simulink model "Test_N3"  (R2022a)
settings: Solver=ode3  StartTime=0.0  StopTime=inf  FixedStep=0.05  RelTol=1e-3
libraries: EcBlockToolbox x1

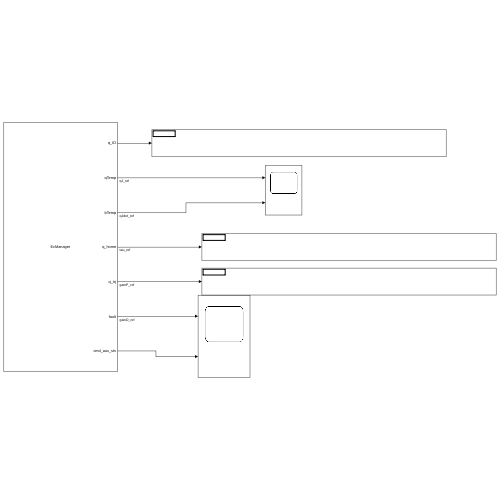
[thumbnail: Simulink's stored preview of the top-level diagram]
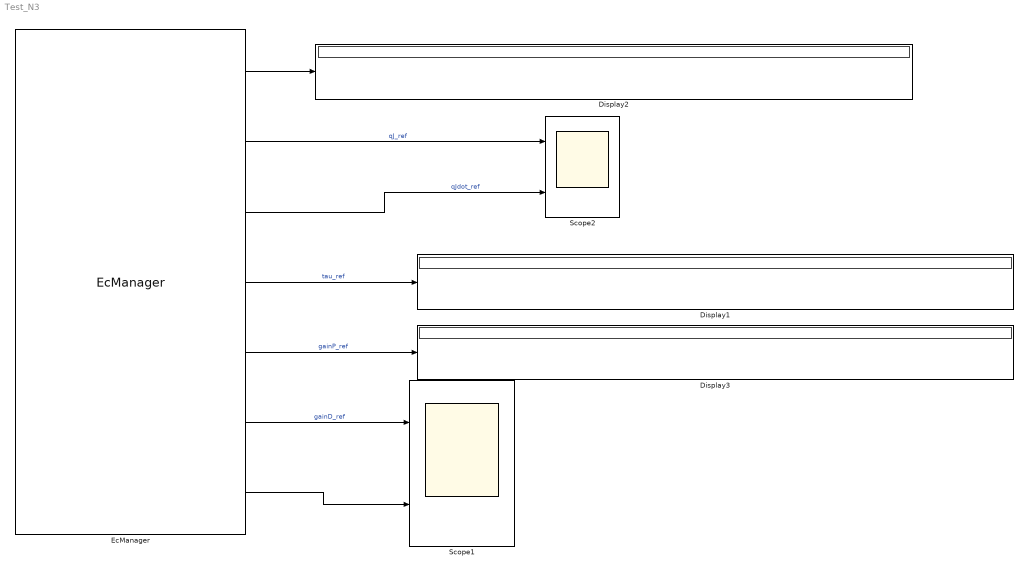
== system Test_N3 ==
  Display1 : Display
  Display2 : Display
  Display3 : Display
  EcManager : EcBlockToolbox/EcManager  PowList={}  ReadingsList={'q_ID', 'qTemp', 'bTemp', 'q_home', 'q_trj', 'fault', 'cmd_aux_sts'}  ReferencesList={}  ImuList={}  FtList={}
  Scope1 : Scope  NumInputPorts=2
  Scope2 : Scope  NumInputPorts=2
  wires:
  EcManager/1 -> Display2/1
  EcManager/2 -> Scope2/1  "qJ_ref"
  EcManager/3 -> Scope2/2  "qJdot_ref"
  EcManager/4 -> Display1/1  "tau_ref"
  EcManager/5 -> Display3/1  "gainP_ref"
  EcManager/6 -> Scope1/1  "gainD_ref"
  EcManager/7 -> Scope1/2
